simulink model "prob1"  (R2018b)
settings: Solver=VariableStepAuto  StartTime=0.0  StopTime=10.0  RelTol=1e-3
values from neighbouring files (symbols this model uses):
  A1 = [0,1;-(k1+k2)/m1,-(c1+c2)/m1]    [exmp1.m]
  B1 = [B11,B12]    [exmp1.m]
  C1 = eye(2)    [exmp1.m]
  D1 = zeros(size(B1,1),size(B1,2))    [exmp1.m]
settings Model: Creator=Hasanlu  LastModifiedBy=Hasanlu

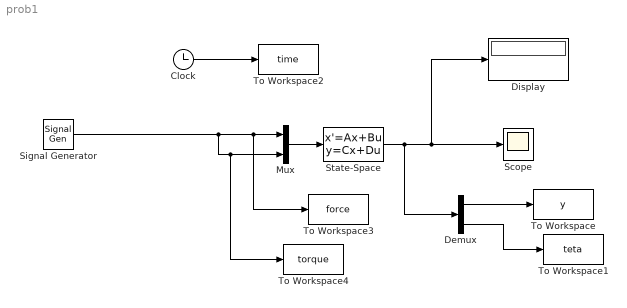
== system prob1 ==
  Clock : Clock
  Demux : Demux  Outputs=2
  Display : Display
  Mux : Mux  Inputs=2
  Scope : Scope
  Signal Generator : SignalGenerator  Frequency=10  Units=rad/sec
  State-Space : StateSpace  A=A1  B=B1  C=C1  D=D1  InitialCondition=0
  To Workspace : ToWorkspace  VariableName=y  SampleTime=-1
  To Workspace1 : ToWorkspace  VariableName=teta  SampleTime=-1
  To Workspace2 : ToWorkspace  VariableName=time  SampleTime=-1
  To Workspace3 : ToWorkspace  VariableName=force  SampleTime=-1
  To Workspace4 : ToWorkspace  VariableName=torque  SampleTime=-1
  wires:
  Mux/1 -> State-Space/1
  State-Space/1 -> Demux/1, Display/1, Scope/1
  Signal Generator/1 -> To Workspace4/1, Mux/2, To Workspace3/1, Mux/1
  Demux/1 -> To Workspace/1
  Demux/2 -> To Workspace1/1
  Clock/1 -> To Workspace2/1
